simulink model "open_loop"  (R2018b)
settings: Solver=VariableStepAuto  StartTime=0.0  StopTime=5  RelTol=1e-3
settings Model: Creator=cnit355  LastModifiedBy=cnit355

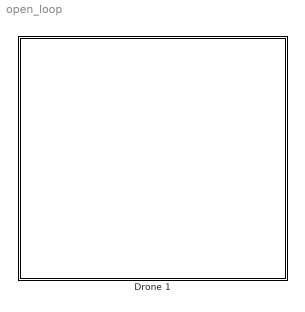
== system open_loop ==
  Drone 1 : Subsystem  Tag=Drone 1

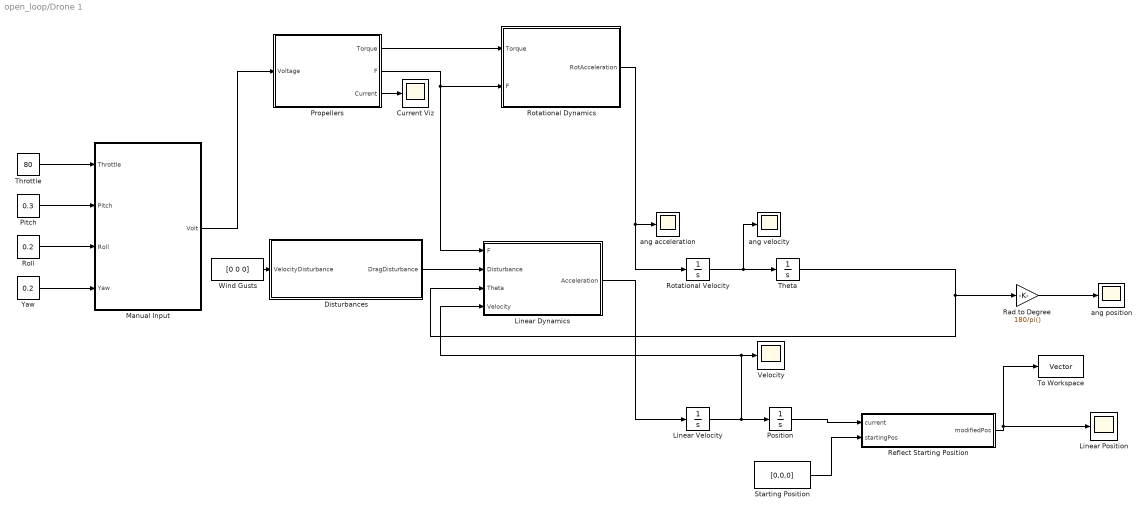
== system open_loop/Drone 1 ==
  Current Viz : Scope
  Disturbances : MATLAB Function  TreatAsAtomicUnit=on
  Linear Dynamics : MATLAB Function  TreatAsAtomicUnit=on
  Linear Position : Scope
  Linear Velocity : Integrator
  Manual Input : MATLAB Function  TreatAsAtomicUnit=on
  Pitch : Constant  Value=0.3
  Position : Integrator
  Propellers : MATLAB Function  TreatAsAtomicUnit=on
  Rad to Degree : Gain  Gain=180/pi()
  Reflect Starting Position : MATLAB Function  TreatAsAtomicUnit=on
  Roll : Constant  Value=0.2
  Rotational Dynamics : MATLAB Function  TreatAsAtomicUnit=on
  Rotational Velocity : Integrator
  Starting Position : Constant  Value=[0,0,0]  VectorParams1D=off
  Theta : Integrator
  Throttle : Constant  Value=80
  To Workspace : ToWorkspace  VariableName=Vector  SampleTime=-1
      settings: Save2DSignal=2-D array (concatenate along first dimension)
  "Velocity " : Scope
  Wind Gusts : Constant  Value=[0 0 0]
  Yaw : Constant  Value=0.2
  ang acceleration : Scope
  "ang position " : Scope
  ang velocity : Scope
  wires:
  Pitch/1 -> Manual Input/2(Pitch)
  Theta/1 -> Linear Dynamics/3(Theta), Rad to Degree/1
  Propellers/3(Current) -> Current Viz/1
  Rotational Velocity/1 -> ang velocity/1, Theta/1
  Linear Velocity/1 -> "Velocity "/1, Linear Dynamics/4(Velocity), Position/1
  Disturbances/1(DragDisturbance) -> Linear Dynamics/2(Disturbance)
  Rotational Dynamics/1(RotAcceleration) -> Rotational Velocity/1, ang acceleration/1
  Rad to Degree/1 -> "ang position "/1
  Linear Dynamics/1(Acceleration) -> Linear Velocity/1
  Manual Input/1(Volt) -> Propellers/1(Voltage)
  Yaw/1 -> Manual Input/4(Yaw)
  Roll/1 -> Manual Input/3(Roll)
  Throttle/1 -> Manual Input/1(Throttle)
  Propellers/1(Torque) -> Rotational Dynamics/1(Torque)
  Propellers/2(F) -> Linear Dynamics/1(F), Rotational Dynamics/2(F)
  Wind Gusts/1 -> Disturbances/1(VelocityDisturbance)
  Position/1 -> Reflect Starting Position/1(current)
  Reflect Starting Position/1(modifiedPos) -> To Workspace/1, Linear Position/1
  Starting Position/1 -> Reflect Starting Position/2(startingPos)

== matlab function open_loop/Drone 1/Rotational Dynamics ==
  data: Torque input; RotAcceleration output; F input
function RotAcceleration = fcn(Torque, F)
Moment = [0 0 0];
RotAcceleration = [0 0 0]; 
Inertia = [0.003, 0.003, 0.007]; %moment of inertia

Moment(1) =  (F(3)+F(4)) * 0.237/2 - (F(1)+F(2))*0.237/2;
Moment(2) =  (F(3)+F(2)) * 0.237/2 - (F(1)+F(4))*0.237/2;
Moment(3) =  Torque(4) - Torque(1) + Torque(2) - Torque(3); %yaw

for i=1:3
    RotAcceleration(i) = Moment(i) / Inertia(i);
end

== matlab function open_loop/Drone 1/Propellers ==
  data: Voltage input; Torque output; F output; Current output
function [Torque, F, Current] = fcn(Voltage)

RPM = [0 0 0 0];
Torque = [0 0 0 0];
Current = [0 0 0 0];
F = [0 0 0 0];

for i=1:4
    RPM(i) = -2.6931*Voltage(i)^3 + 1400*Voltage(i);
    Ct = 2 * (10^-15) * (RPM(i)^3) - 4 * (10^-11) * (RPM(i)^2) + 3 * (10^(-7)) * RPM(i) + 0.1013;
    F(i) = Ct * 1.225*(RPM(i)/60)^2 * 0.2^4; %0.2 = diameter of propeller
    Torque(i) = 4 * 10^-14 * RPM(i)^3 + 8 * 10^-12 * RPM(i)^2 + 3 * 10^-6 * RPM(i);
    Current(i) = 1400*Torque(i);
end

== matlab function open_loop/Drone 1/Linear Dynamics ==
  data: F input; Acceleration output; Disturbance input; Theta input; Velocity input
function Acceleration  = fcn(F,Disturbance,Theta,Velocity)
m=0.743; %mass
g=9.81; %gravity
A=[0.0197 0.0197 0.0512]; %projected area 
air=1.225; %air density
Cd=1; %coefficient of drag

Acceleration=[0 0 0];
Force = [0 0 0];
Fprop = [0 0 0]; %thrust in x,y,z direction
% Prop=[0;0;0];

Fprop(1)=sin(Theta(2))*cos(Theta(1))*(F(1)+F(2)+F(3)+F(4));
Fprop(2)=sin(Theta(1))*cos(Theta(2))*(F(1)+F(2)+F(3)+F(4));
Fprop(3)=cos(Theta(1))*cos(Theta(2))*(F(1)+F(2)+F(3)+F(4));
% Prop(1,1)=sin(Theta(2))*cos(Theta(1))*(F(1)+F(2)+F(3)+F(4));
% Prop(2,1)=sin(Theta(1))*cos(Theta(2))*(F(1)+F(2)+F(3)+F(4));
% Prop(3,1)=(F(1)+F(2)+F(3)+F(4))*cos(Theta(1))*cos(Theta(2));

ThetaXY = -atan2(Fprop(1),Fprop(2));
XY2D=sqrt(Fprop(1)^2+Fprop(2)^2); %thrust projection vector

%Yaw 
if Fprop(3)>=0
    Fprop(1)=XY2D*sin(Theta(3)+ThetaXY); %magnitude of 2d vector * sign(angle + yaw motion)
    Fprop(2)=XY2D*cos(Theta(3)+ThetaXY);
else
     Fprop(1)=XY2D*sin(-Theta(3)+ThetaXY);
    Fprop(2)=XY2D*cos(-Theta(3)+ThetaXY);
end

%+ - drag based on move forward/ backward
if Velocity(1)<0
    Force(1)=Fprop(1)-Disturbance(1)+0.5*air*Velocity(1)^2*A(1)*Cd;
else 
    Force(1)=Fprop(1)-Disturbance(1)-0.5*air*Velocity(1)^2*A(1)*Cd;
end

if Velocity(2)<0
    Force(2)=Fprop(2)-Disturbance(2)+0.5*air*Velocity(2)^2*A(2)*Cd;
else 
    Force(2)=Fprop(2)-Disturbance(2)-0.5*air*Velocity(2)^2*A(2)*Cd;
end

if Velocity(3)<0
    Force(3)=Fprop(3)+0.5*air*Velocity(3)^2*A(3)*Cd-m*g-Disturbance(3);
else 
    Force(3)=Fprop(3)-0.5*air*Velocity(3)^2*A(3)*Cd-m*g-Disturbance(3);
end

disp("FORCE")
disp(Force)
for i=1:3
    Acceleration(i)=Force(i)/m;
end

== matlab function open_loop/Drone 1/Disturbances ==
  data: VelocityDisturbance input; DragDisturbance output
function DragDisturbance = fcn(VelocityDisturbance)
A=[0.0197 0.0197 0.0197*2*1.3]; %x,y,z direction
DragDisturbance=[0 0 0];
rho=1.225; %sea level
Cd=1; %coefficient of drag

for i=1:3
    if VelocityDisturbance(i) < 0
        DragDisturbance(i)= 0.5*rho*VelocityDisturbance(i)^2*A(i)*Cd;
    else
        DragDisturbance(i)= -0.5*rho*VelocityDisturbance(i)^2*A(i)*Cd;
    end
end

== matlab function open_loop/Drone 1/Manual Input ==
  data: Throttle input; Volt output; Pitch input; Roll input; Yaw input
function Volt = fcn(Throttle, Pitch, Roll, Yaw)

Correct = 0; %correction of final voltage
%increase, decrease throttle level that symmetry works

%condition of each input 
%Throttle <- increase and decrease pitch roll yaw symetrically
if (Pitch/2+Roll/2+Yaw/2) > (100-Throttle) % -50 ~ +50
   
    Correct = ((Pitch/2 + Roll/2 + Yaw/2) - (100 - Throttle));
       
end

if Throttle > 10 && (Pitch/2+Roll/2+Yaw/2) > (Throttle-10) %Enough space for other size // make it never go down to 10%... -10 will result in false movement

    if Correct < ((Pitch/2 + Roll/2 + Yaw/2) - (Throttle - 10)) % jf too big, take excess
        Correct = ((Pitch/2 + Roll/2 + Yaw/2) - (Throttle - 10)) ;   
    end
            
end

if Correct ~= 0 
    %Correct pitch, roll, yaw from user input
    Pitch = Pitch - Correct / 3 * 2; %distribute excess to pitch, roll, and yaw
    Roll = Roll - Correct / 3 * 2;
    Yaw = Yaw - Correct / 3 * 2;
end

%voltage for each motor
Volt = [(Throttle - Pitch / 2 - Roll / 2 - Yaw / 2)*11.4/100 %percent=> divide by 100 /  voltage max = 11.4
    (Throttle - Pitch / 2 + Roll / 2 + Yaw / 2)*11.4/100
    (Throttle + Pitch / 2 + Roll / 2 - Yaw / 2)*11.4/100
    (Throttle + Pitch / 2 - Roll / 2 + Yaw / 2)*11.4/100];

== matlab function open_loop/Drone 1/Reflect Starting Position ==
  data: current input; modifiedPos output; startingPos input
function modifiedPos = fcn(current, startingPos)
disp(current)
disp(startingPos)
modifiedPos = current + startingPos;
